simulink model "Copy_of_exam3_sim_2"  (R2023a)
settings: Solver=VariableStepAuto  StartTime=0.0  StopTime=4  FixedStep=sim_step  RelTol=1e-3
values from neighbouring files (symbols this model uses):
  B = 0.0024    [8_21_oct16.mat]    (also in 8_26_oct16.mat; 9_00_oct16_param_wkb.mat; I-PD_pid.mat; exam3.m)
  J_m = 0.005    [8_21_oct16.mat]    (also in 8_26_oct16.mat; 9_00_oct16_param_wkb.mat; I-PD_pid.mat; exam3.m)
  k_d = 0.270673740678    [8_21_oct16.mat]    (also in 8_26_oct16.mat = 0.547706203354; 9_00_oct16_param_wkb.mat = 0.258677937097; I-PD_pid.mat = 0.165462892088)
  k_i = 1.2879299488    [8_21_oct16.mat]    (also in 8_26_oct16.mat = 1.24340964176; 9_00_oct16_param_wkb.mat = 1.541738552; I-PD_pid.mat = 30; exam3.m = 0.4673766)
  k_p = 4.15772580161    [8_21_oct16.mat]    (also in 8_26_oct16.mat = 9.26358212797; 9_00_oct16_param_wkb.mat = 3.36920723092; I-PD_pid.mat = 3.40616838103; exam3.m = 2.16754540129)
  M_n = 6.4    [8_21_oct16.mat]    (also in 8_26_oct16.mat; 9_00_oct16_param_wkb.mat; I-PD_pid.mat; exam3.m)
  Nel = 10000    [8_21_oct16.mat]    (also in 8_26_oct16.mat; 9_00_oct16_param_wkb.mat; I-PD_pid.mat; exam3.m)
  T_n = 0.015    [8_21_oct16.mat]    (also in 8_26_oct16.mat; 9_00_oct16_param_wkb.mat; I-PD_pid.mat; exam3.m)
  Tvz = 0.004    [8_21_oct16.mat]    (also in 8_26_oct16.mat; 9_00_oct16_param_wkb.mat; I-PD_pid.mat; exam3.m)
undefined symbols (not defined in the file or in its folder): DiscIntNeverNeededParam, k_i_s, k_p_s
libraries: simulink x1, SignalEditorBlockLib x1
settings Model: Creator=laptop  LastModifiedBy=laptop

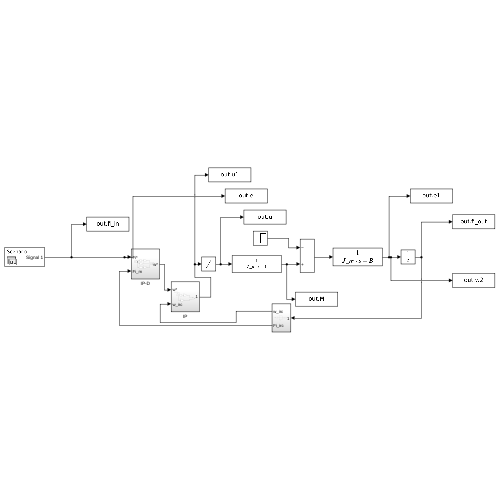
[thumbnail: Simulink's stored preview of the top-level diagram]
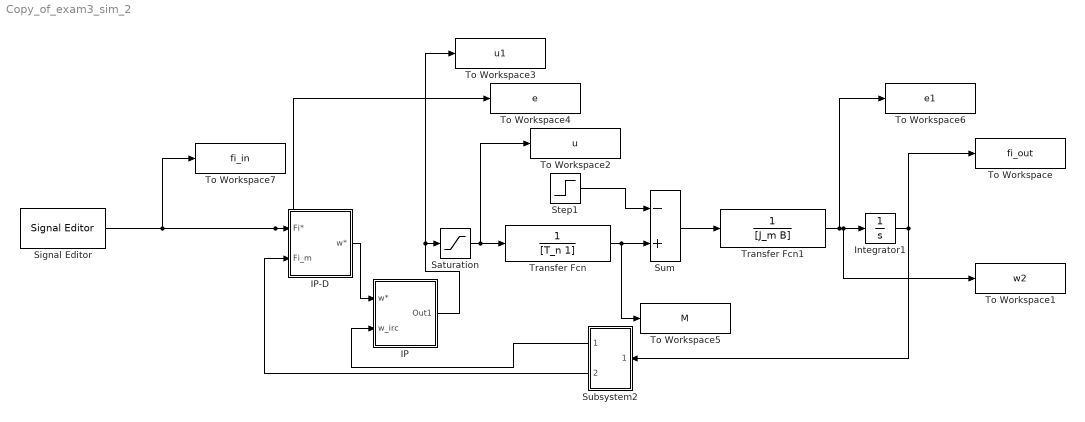
== system Copy_of_exam3_sim_2 ==
  IP : Subsystem
  IP-D : Subsystem
  Integrator1 : Integrator
  Saturation : Saturate  UpperLimit=M_n*0.75  LowerLimit=-M_n*0.75
  Signal Editor : SignalEditorBlockLib/Signal Editor  FileName=signalmat.mat  ActiveScenario=Scenario  ActiveSignal=Signal 1  IsBus=off  OutputBusObjectStr=Bus: BusObject  SampleTime=0  Interpolate=off  ZeroCross=off  OutputAfterFinalValue=Holding final value  Unit=inherit  PreserveSignalName=on  ApplySigPropsToAllScenarios=on
  Step1 : Step  After=M_n*0.1  SampleTime=0
  Subsystem2 : Subsystem
  Sum : Sum  Inputs=-+
  To Workspace : ToWorkspace  VariableName=fi_out  SaveFormat=Timeseries  SampleTime=-1
  To Workspace1 : ToWorkspace  VariableName=w2  SaveFormat=Timeseries  SampleTime=-1
  To Workspace2 : ToWorkspace  VariableName=u  SaveFormat=Timeseries  SampleTime=-1
  To Workspace3 : ToWorkspace  VariableName=u1  SaveFormat=Timeseries  SampleTime=-1
  To Workspace4 : ToWorkspace  VariableName=e  SaveFormat=Timeseries  SampleTime=-1
  To Workspace5 : ToWorkspace  VariableName=M  SaveFormat=Timeseries  SampleTime=-1
  To Workspace6 : ToWorkspace  VariableName=e1  SaveFormat=Timeseries  SampleTime=-1
  To Workspace7 : ToWorkspace  VariableName=fi_in  SaveFormat=Timeseries  SampleTime=-1
  Transfer Fcn : TransferFcn  Denominator=[T_n 1]
  Transfer Fcn1 : TransferFcn  Denominator=[J_m B]
  wires:
  Transfer Fcn/1 -> To Workspace5/1, Sum/2
  Saturation/1 -> Transfer Fcn/1, To Workspace2/1
  Sum/1 -> Transfer Fcn1/1
  Transfer Fcn1/1 -> To Workspace6/1, To Workspace1/1, Integrator1/1
  Step1/1 -> Sum/1
  Integrator1/1 -> Subsystem2/1(In1), To Workspace/1
  Signal Editor/1 -> To Workspace4/1, IP-D/1(Fi*), To Workspace7/1
  Subsystem2/2(Fi_irc) -> IP-D/2(Fi_m)
  IP/1(Out1) -> To Workspace3/1, Saturation/1
  IP-D/1(w*) -> IP/1(w*)
  Subsystem2/1(w_irc) -> IP/2(w_irc)

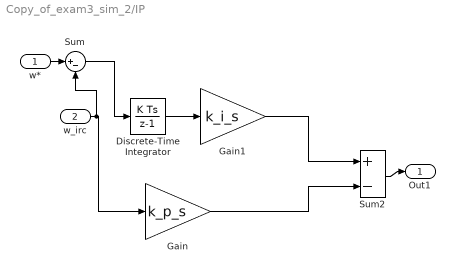
== system Copy_of_exam3_sim_2/IP ==
  w* : Inport
  w_irc : Inport  Port=2
  Discrete-Time Integrator : DiscreteIntegrator  SampleTime=Tvz  ICPrevOutput=DiscIntNeverNeededParam  ICPrevScaledInput=DiscIntNeverNeededParam
  Gain : Gain  Gain=k_p_s
  Gain1 : Gain  Gain=k_i_s
  Sum : Sum  Inputs=|+-
  Sum2 : Sum  Inputs=+-
  Out1 : Outport
  wires:
  Discrete-Time Integrator/1 -> Gain1/1
  Gain/1 -> Sum2/2
  Sum2/1 -> Out1/1
  w_irc/1 -> Gain/1, Sum/2
  Gain1/1 -> Sum2/1
  w*/1 -> Sum/1
  Sum/1 -> Discrete-Time Integrator/1

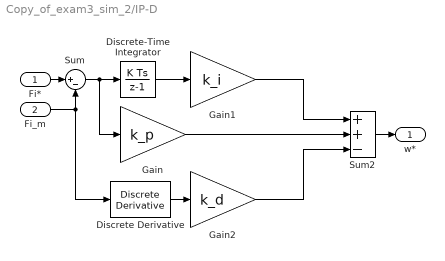
== system Copy_of_exam3_sim_2/IP-D ==
  Fi* : Inport
  Fi_m : Inport  Port=2
  Discrete Derivative : simulink/Discrete/Discrete Derivative  gainval=1.0  ICPrevScaledInput=0.0  OutMin=[]  OutMax=[]  OutDataType=fixdt(1, 16)  OutScaling=2^-10  DoSatur=off
  Discrete-Time Integrator : DiscreteIntegrator  SampleTime=Tvz  ICPrevOutput=DiscIntNeverNeededParam  ICPrevScaledInput=DiscIntNeverNeededParam
  Gain : Gain  Gain=k_p
  Gain1 : Gain  Gain=k_i
  Gain2 : Gain  Gain=k_d
  Sum : Sum  Inputs=|+-
  Sum2 : Sum  Inputs=++-
  w* : Outport
  wires:
  Discrete-Time Integrator/1 -> Gain1/1
  Gain2/1 -> Sum2/3
  Discrete Derivative/1 -> Gain2/1
  Gain/1 -> Sum2/2
  Sum2/1 -> w*/1
  Gain1/1 -> Sum2/1
  Fi*/1 -> Sum/1
  Fi_m/1 -> Discrete Derivative/1, Sum/2
  Sum/1 -> Gain/1, Discrete-Time Integrator/1

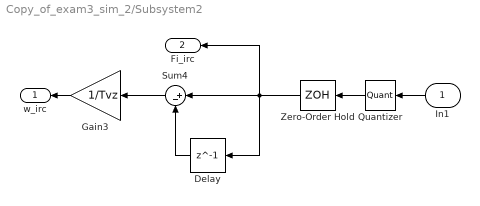
== system Copy_of_exam3_sim_2/Subsystem2 ==
  In1 : Inport
  Delay : Delay  DelayLength=1
  Gain3 : Gain  Gain=1/Tvz
  Quantizer : Quantizer  QuantizationInterval=2*pi/Nel
  Sum4 : Sum  Inputs=|+-
  Zero-Order Hold : ZeroOrderHold  SampleTime=Tvz
  w_irc : Outport
  Fi_irc : Outport  Port=2
  wires:
  Sum4/1 -> Gain3/1
  Delay/1 -> Sum4/2
  Zero-Order Hold/1 -> Delay/1, Sum4/1, Fi_irc/1
  In1/1 -> Quantizer/1
  Quantizer/1 -> Zero-Order Hold/1
  Gain3/1 -> w_irc/1
